simulink model "thermal_subsystem_closed_loop_harness"  (R2023a)
settings: Solver=VariableStepAuto  StartTime=0.0  StopTime=600  RelTol=1e-3
PostLoadFcn:
  | run('thermal_subsystem_parameters.m')
  | run('thermal_subsytem_harness_parameters.m')
values from neighbouring files (symbols this model uses):
  coolant_initial_temperature = 293.15    [thermal_model_parameters.m]    (also in thermal_plant_h2f175_parameters.m)
undefined symbols (not defined in the file or in its folder): sigbuilder_block, stack
libraries: fl_lib x5, nesl_utility x3, simulink x1
settings Model: Creator=adrian.taveras  LastModifiedBy=stefan.notter
settings OptimizationCC: ReuseModelBlockBuffer=off

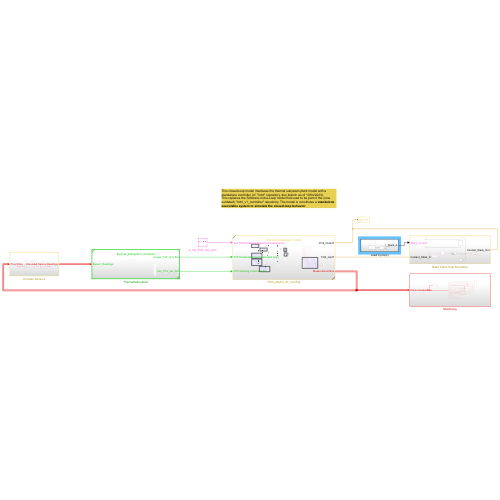
[thumbnail: Simulink's stored preview of the top-level diagram]
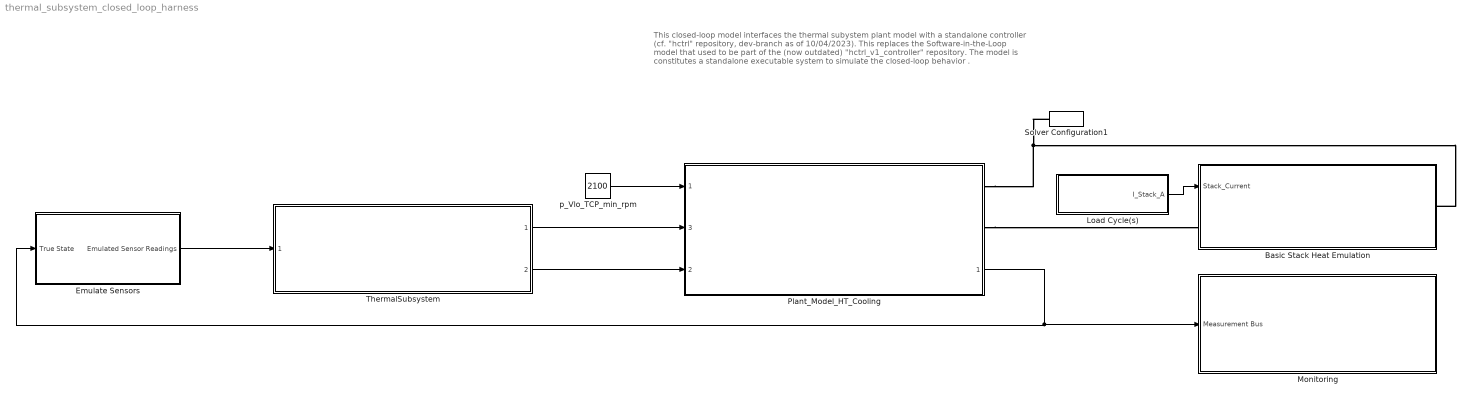
== system thermal_subsystem_closed_loop_harness ==
  note: This closed-loop model interfaces the thermal subystem plant model with a standalone controller (cf. "hctrl" repository, dev-branch as of 10/04/2023).
      | This replaces the Software-in-the-Loop model that used to be part of the (now outdated) "hctrl_v1_controller" repository. The model is constitutes a standalone executable system to simulate the closed-loop behavior .
  Basic Stack Heat Emulation : Subsystem
  Emulate Sensors : Subsystem
  Load Cycle(s) : Subsystem
  Monitoring : Subsystem
  Plant_Model_HT_Cooling : Subsystem  ReferencedSubsystem=thermal_subsystem_model
      settings: PortSchema="{\"entries\":[{\"content\":{\"sides\":[{\"content\":{\"connectorIds\":[\"Out1\",\"LConn1\",\"LConn2\"]},\"type\":\"ConnectorPlacement.EquallySpacedRectSide\",\"uuid\":\"706cf171-be05-45fb-992c-ba5e90f5cdb8\"},{\"content\":{\"connectorIds\":[\"In2\",\"In3\",\"In1\"],\"side\":\"RIGHT\"},\"type\":\"ConnectorPlacement.EquallySpacedRectSide\",\"uuid\":\"bf8ca14f-fef4-4eb5-a927-ccc799898aca\"},{\"content\":{\"side\":\"TOP\"},\"type\":\"ConnectorPlacement.EquallySpacedRectSide\",\"uuid\":\"9ad70fe7-ae85-4ea7-9728-0856e6ff40bf\"}]},\"type\":\"ConnectorPlacement.EquallySpacedConnector\",\"uuid\":\"91c985a6-7405-42c3-ac14-8c35e74d3001\"}],\"packageUris\":[\"http://schema.mathworks.com/mf0/Connector/R2020b\"],\"version\":\"1.0\"}"
  Solver Configuration1 : nesl_utility/Solver Configuration  PhysicalDomain=network_engine_domain  SubClassName=solver  LeftPortType=input  RightPortType=generic  Tones=[]  Harmonics=[]  SimulateNoise=off  Profile=off  UseLocalSampling=off  EnableSwitchedLinearOptims=on  FrequencyDomain=off  UseCCode=off  RelTol=0.001  AbsTol=1e-06  MinStep=1e-09  ToWorkspace=off  RevertToSquareIcSolve=off  NumHomotopyIterations=100  PhasorMode=off  PhasorModeNumHarmonics=1  ConsistencySolver=NEWTON_XTOL_AFTER_FTOL  IndexReductionMethod=DerivativeReplacement  DoDC=off  ResidualTolerance=1e-09  ConsistencyTolSource=GLOBAL  ConsistencyAbsTol=0.001  ConsistencyRelTol=0.001  ConsistencyTolFactor=0.001  UseLocalSolver=on  LocalSolverChoice=NE_BACKWARD_EULER_ADVANCER  ResolveIndetEquations=on  FunctionEvalNumThread=1  LocalSolverSampleTime=0.001  DoFixedCost=on  MaxNonlinIter=3  MaxModeIter=2  ComputeImpulses=off  ImpulseIterations=2  LinearAlgebra=auto  LinearAlgebraNumThread=0  EquationFormulation=NE_TIME_EF  DelaysMemoryBudget=1024  AutomaticFiltering=off  FilteringTimeConstant=0.001  PartitionStorageMethod=AS_NEEDED  PartitionMemoryBudget=1024  PartitionMethod=ROBUST
  ThermalSubsystem : Subsystem  TreatAsAtomicUnit=on  SystemSampleTime=0.02  ReferencedSubsystem=thermal_subsystem_controller
      settings: RTWFcnNameOpts=Use subsystem name  RTWFileNameOpts=Use subsystem name
  p_Vlo_TCP_min_rpm : Constant  Value=2100
  wires:
  Plant_Model_HT_Cooling/1 -> Emulate Sensors/1(True State), Monitoring/1(Measurement Bus)
  Emulate Sensors/1(Emulated Sensor Readings) -> ThermalSubsystem/1
  ThermalSubsystem/1 -> Plant_Model_HT_Cooling/3
  p_Vlo_TCP_min_rpm/1 -> Plant_Model_HT_Cooling/1
  ThermalSubsystem/2 -> Plant_Model_HT_Cooling/2
  Load Cycle(s)/1(I_Stack_A) -> Basic Stack Heat Emulation/1(Stack_Current)
  connections:
  Plant_Model_HT_Cooling/LConn1 -- Basic Stack Heat Emulation/LConn1
  Plant_Model_HT_Cooling/LConn2 -- Solver Configuration1/RConn1 -- Basic Stack Heat Emulation/RConn1

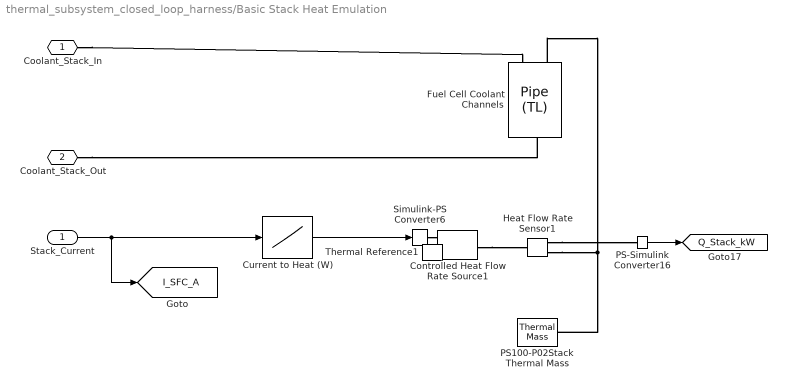
== system thermal_subsystem_closed_loop_harness/Basic Stack Heat Emulation ==
  Stack_Current : Inport
  Controlled Heat Flow Rate Source1 : fl_lib/Thermal/Thermal Sources/Controlled Heat Flow Rate Source
  Current to Heat (W) : Lookup_n-D  NumberOfTableDimensions=1  BreakpointsForDimension1=[0:50:400]  Table=[0, 9932, 21438, 33442,47123, 59491, 77033, 93585, 112042]  InternalRulePriority=Speed  RndMeth=Simplest
  Fuel Cell Coolant Channels : fl_lib/Thermal Liquid/Elements/Pipe (TL)  length=sqrt(stack.area) * stack.coolant_num_passes cm  area=stack.coolant_w_channels^2 * stack.coolant_num_layers cm^2  Dh=stack.coolant_w_channels cm  length_add=10 cm  roughness=15e-5 m  Re_lam=2000  Re_tur=4000  shape_factor=64  Nu_lam=3.66  dynamic_compressibility=simscape.enum.onoff.on  inertia=simscape.enum.onoff.off  p0=coolant_initial_pressure MPa  T0=coolant_initial_temperature K  mdot0=0 kg/s
  Heat Flow Rate Sensor1 : fl_lib/Thermal/Thermal Sensors/Heat Flow Rate Sensor
  PS-Simulink Converter16 : nesl_utility/PS-Simulink Converter  PhysicalDomain=network_engine_domain  SubClassName=ps_output  LeftPortType=input  RightPortType=output  PseudoPeriodic=off  Frequencies=[]  VectorFormat=1-D array  Unit=kW  AffineConversion=off
  PS100-P02Stack Thermal Mass : fl_lib/Thermal/Thermal Elements/Thermal Mass  mass_type=foundation.enum.constant_variable.constant  mass=stack.thermal_mass kg  sp_heat=stack.specific_heat J/kg/K  mass_min=1e-6 kg  num_ports=foundation.enum.numPorts2.one  m_specify=off  m_priority=High  m=1 kg  m_nominal_specify=off  m_nominal_unit=kg  m_nominal_value=1  T_specify=on  T_priority=High  T=coolant_initial_temperature K  T_nominal_specify=off  T_nominal_unit=K  T_nominal_value=1  Q_specify=off  Q_priority=None  Q=20e3 W  Q_nominal_specify=off  Q_nominal_unit=W  Q_nominal_value=1
  Simulink-PS Converter6 : nesl_utility/Simulink-PS Converter  PhysicalDomain=network_engine_domain  SubClassName=ps_input  LeftPortType=input  RightPortType=output  PseudoPeriodic=off  Frequencies=[]  NoiseDistribution=none  NoiseParameters=[]  Unit=J/s  AffineConversion=off  FilteringAndDerivatives=provide  SimscapeFilterOrder=1  InputFilterTimeConstant=0.001  UdotUserProvided=0
  Thermal Reference1 : fl_lib/Thermal/Thermal Elements/Thermal Reference
  Coolant_Stack_Out : PMIOPort  Port=2  Side=Right
  Coolant_Stack_In : PMIOPort  Side=Left
  tag scope: I_SFC_A=global, Q_Stack_kW=global
  wires:
  Current to Heat (W)/1 -> Simulink-PS Converter6/1
  PS-Simulink Converter16/1 -> [Q_Stack_kW]
  Stack_Current/1 -> Current to Heat (W)/1, [I_SFC_A]
  connections:
  Thermal Reference1/LConn1 -- Controlled Heat Flow Rate Source1/RConn2
  Controlled Heat Flow Rate Source1/LConn1 -- Heat Flow Rate Sensor1/LConn1
  Fuel Cell Coolant Channels/LConn2 -- Heat Flow Rate Sensor1/RConn2 -- PS100-P02Stack Thermal Mass/LConn1
  Heat Flow Rate Sensor1/RConn1 -- PS-Simulink Converter16/LConn1
  Simulink-PS Converter6/RConn1 -- Controlled Heat Flow Rate Source1/RConn1
  Coolant_Stack_In/RConn1 -- Fuel Cell Coolant Channels/LConn1
  Coolant_Stack_Out/RConn1 -- Fuel Cell Coolant Channels/RConn1

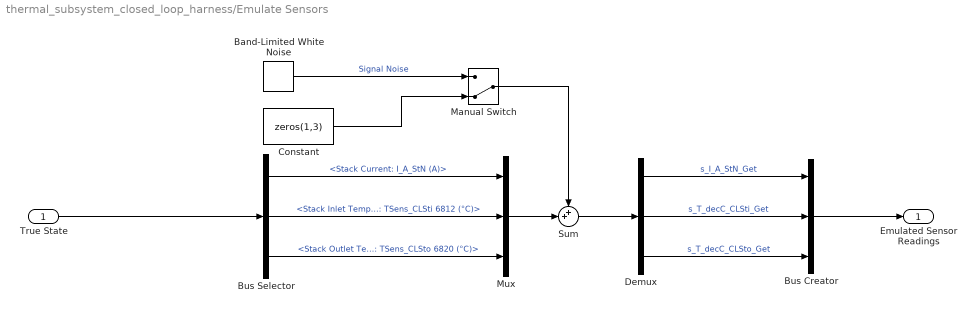
== system thermal_subsystem_closed_loop_harness/Emulate Sensors ==
  True State : Inport
  Band-Limited White Noise : simulink/Sources/Band-Limited White Noise  Cov=[5e-3, 5e-4, 5e-4]  Ts=0.1  seed=[23341]
  Bus Creator : BusCreator  Inputs=3
  Bus Selector : BusSelector  OutputSignals=Stack Current: I_A_StN (A),Stack Inlet Temperature: TSens_CLSti 6812 (°C),Stack Outlet Temperature: TSens_CLSto 6820 (°C)
  Constant : Constant  Value=zeros(1,3)
  Demux : Demux  Outputs=3
  Manual Switch : ManualSwitch  CurrentSetting=0
  Mux : Mux  Inputs=3
  Sum : Sum  Inputs=++|
  Emulated Sensor Readings : Outport
  wires:
  Bus Creator/1 -> Emulated Sensor Readings/1
  True State/1 -> Bus Selector/1
  Bus Selector/1 -> Mux/1  "<Stack Current: I_A_StN (A)>"
  Bus Selector/2 -> Mux/2  "<Stack Inlet Temperature: TSens_CLSti 6812 (°C)>"
  Bus Selector/3 -> Mux/3  "<Stack Outlet Temperature: TSens_CLSto 6820 (°C)>"
  Mux/1 -> Sum/2
  Sum/1 -> Demux/1
  Manual Switch/1 -> Sum/1
  Band-Limited White Noise/1 -> Manual Switch/1  "Signal Noise"
  Constant/1 -> Manual Switch/2
  Demux/1 -> Bus Creator/1  "s_I_A_StN_Get"
  Demux/3 -> Bus Creator/3  "s_T_decC_CLSto_Get"
  Demux/2 -> Bus Creator/2  "s_T_decC_CLSti_Get"

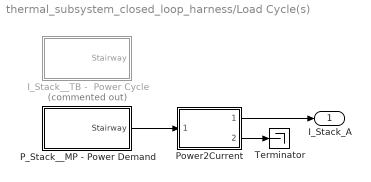
== system thermal_subsystem_closed_loop_harness/Load Cycle(s) ==
  I_Stack__TB -  Power Cycle : Subsystem  Tag=STV Subsys  Commented=on  LoadFcn=sigbuilder_block('load');  StartFcn=sigbuilder_block('start');  StopFcn=sigbuilder_block('stop');  ClipboardFcn=sigbuilder_block('clipboard');  mask(Sigbuilder block){tuvar=[0:10]}
      mask help: Simulink:masks:SigbuilderBlock_MD
      mask init:
      | if ~strcmp(get_param(bdroot(gcbh),'SimulationStatus'),'stopped') tuvar = sigbuilder_block('maskInit'); end
      settings: CopyFcn=sigbuilder_block('copy');  DeleteFcn=sigbuilder_block('delete');  ModelCloseFcn=sigbuilder_block('modelClose');  PreSaveFcn=sigbuilder_block('preSave');  PauseFcn=sigbuilder_block('pause');  ContinueFcn=sigbuilder_block('continue');  NameChangeFcn=sigbuilder_block('namechange');  OpenFcn=sigbuilder_block('open',[150.6 139.8 551.4 322.2 ]);  CloseFcn=sigbuilder_block('close');
      mask Display: plot(0, 0, 100, 100,[2, 2, 32, 32, 2], [68, 8, 8, 68, 68],[32, 2], [38, 38], [32, 19, 2],[53, 60, 44], [32, 17, 17, 2],[16, 16, 31, 31]);txt = getActiveGroup(gcbh);text(2, 100, txt,'verticalAlignment', 'top');
  P_Stack__MP - Power Demand : Subsystem  Tag=STV Subsys  LoadFcn=sigbuilder_block('load');  StartFcn=sigbuilder_block('start');  StopFcn=sigbuilder_block('stop');  ClipboardFcn=sigbuilder_block('clipboard');  mask(Sigbuilder block){tuvar=[0:10]}
      mask help: Simulink:masks:SigbuilderBlock_MD
      mask init:
      | if ~strcmp(get_param(bdroot(gcbh),'SimulationStatus'),'stopped') tuvar = sigbuilder_block('maskInit'); end
      settings: CopyFcn=sigbuilder_block('copy');  DeleteFcn=sigbuilder_block('delete');  ModelCloseFcn=sigbuilder_block('modelClose');  PreSaveFcn=sigbuilder_block('preSave');  PauseFcn=sigbuilder_block('pause');  ContinueFcn=sigbuilder_block('continue');  NameChangeFcn=sigbuilder_block('namechange');  OpenFcn=sigbuilder_block('open',[5.4 5.4 1141.2 580.8 ]);  CloseFcn=sigbuilder_block('close');
      mask Display: plot(0, 0, 100, 100,[2, 2, 32, 32, 2], [68, 8, 8, 68, 68],[32, 2], [38, 38], [32, 19, 2],[53, 60, 44], [32, 17, 17, 2],[16, 16, 31, 31]);txt = getActiveGroup(gcbh);text(2, 100, txt,'verticalAlignment', 'top');
  Power2Current : Subsystem
  Terminator : Terminator
  I_Stack_A : Outport
  wires:
  P_Stack__MP - Power Demand/1(Stairway) -> Power2Current/1(P_Stack)
  Power2Current/2(V_Stack) -> Terminator/1
  Power2Current/1(I_Stack) -> I_Stack_A/1

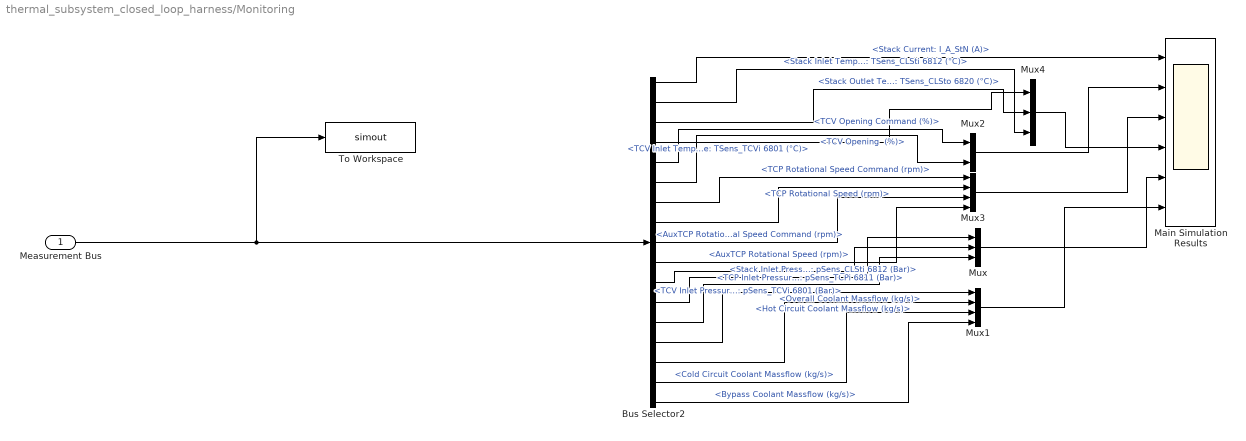
== system thermal_subsystem_closed_loop_harness/Monitoring ==
  Measurement Bus : Inport
  Bus Selector2 : BusSelector  OutputSignals="Stack Current: I_A_StN (A),Stack Inlet Temperature: TSens_CLSti 6812 (°C),Stack Outlet Temperature: TSens_CLSto 6820 (°C),TCV Inlet Temperature: TSens_TCVi 6801 (°C),TCV Opening Command (%),TCV Opening  (%),TCP Rotational Speed Command (rpm),TCP Rotational Speed (rpm),AuxTCP Rotational Speed Command (rpm),AuxTCP Rotational Speed (rpm),TCP Inlet Pressure: pSens_TCPi 6811 (Bar),Stack Inlet Pressure: pSens_CLSti 6812 (Bar),TCV Inlet Pressure: pSens_TCVi 6801 (Bar),Overall Coolant Massflow (kg/s),Hot Circuit Coolant Massflow (kg/s),Cold Circuit Coolant Massflow (kg/s),Bypass Coolant Massflow (kg/s)"
  Main Simulation Results : Scope  NumInputPorts=6
  Mux : Mux  Inputs=3
  Mux1 : Mux
  Mux2 : Mux  Inputs=2
  Mux3 : Mux
  Mux4 : Mux  Inputs=3
  To Workspace : ToWorkspace  VariableName=simout  SaveFormat=Timeseries  SampleTime=-1
  wires:
  Bus Selector2/10 -> Mux3/4  "<AuxTCP Rotational Speed (rpm)>"
  Mux4/1 -> Main Simulation Results/4
  Bus Selector2/11 -> Mux/2  "<TCP Inlet Pressure: pSens_TCPi 6811 (Bar)>"
  Mux3/1 -> Main Simulation Results/3
  Bus Selector2/7 -> Mux3/1  "<TCP Rotational Speed Command (rpm)>"
  Bus Selector2/3 -> Mux4/2  "<Stack Outlet Temperature: TSens_CLSto 6820 (°C)>"
  Mux2/1 -> Main Simulation Results/2
  Measurement Bus/1 -> To Workspace/1, Bus Selector2/1
  Bus Selector2/9 -> Mux3/3  "<AuxTCP Rotational Speed Command (rpm)>"
  Bus Selector2/2 -> Mux4/3  "<Stack Inlet Temperature: TSens_CLSti 6812 (°C)>"
  Bus Selector2/6 -> Mux2/2  "<TCV Opening  (%)>"
  Mux/1 -> Main Simulation Results/5
  Bus Selector2/15 -> Mux1/2  "<Hot Circuit Coolant Massflow (kg/s)>"
  Bus Selector2/13 -> Mux/3  "<TCV Inlet Pressure: pSens_TCVi 6801 (Bar)>"
  Bus Selector2/14 -> Mux1/1  "<Overall Coolant Massflow (kg/s)>"
  Mux1/1 -> Main Simulation Results/6
  Bus Selector2/17 -> Mux1/4  "<Bypass Coolant Massflow (kg/s)>"
  Bus Selector2/8 -> Mux3/2  "<TCP Rotational Speed (rpm)>"
  Bus Selector2/5 -> Mux2/1  "<TCV Opening Command (%)>"
  Bus Selector2/16 -> Mux1/3  "<Cold Circuit Coolant Massflow (kg/s)>"
  Bus Selector2/12 -> Mux/1  "<Stack Inlet Pressure: pSens_CLSti 6812 (Bar)>"
  Bus Selector2/4 -> Mux4/1  "<TCV Inlet Temperature: TSens_TCVi 6801 (°C)>"
  Bus Selector2/1 -> Main Simulation Results/1  "<Stack Current: I_A_StN (A)>"

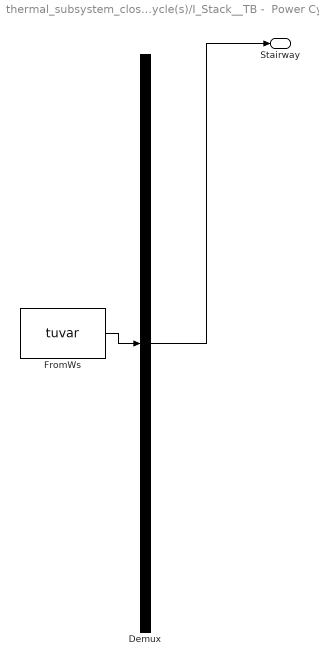
== system thermal_subsystem_closed_loop_harness/Load Cycle(s)/I_Stack__TB -  Power Cycle ==
  Demux : Demux  Tag=STV Demux  Outputs=1
      settings: DisplayOption=none
  FromWs : FromWorkspace  Tag=STV FromWs  VariableName=tuvar
      SigBuilderData=|
      | common.afterFinalStr = 'Extrapolate'
      | common.sampleTime = 0
      | dataSet.timeRange = [0 600]
      | dataSet.name = 'Group 1'
      | sbobj.Groups.Name = 'Group 1'
      | sbobj.Groups.Signals.Name = 'Stairway'
      | sbobj.Groups.Signals.XData = [0 180 190 250 260 320 330 390 400 460 470 530 540 600]
      | sbobj.Groups.Signals.YData = [100 100 200 200 300 300 400 400 300 300 200 200 100 100]
      | sbobj.Groups.TimeRange = [0 600]
  Stairway : Outport  Tag=STV Outport
  wires:
  Demux/1 -> Stairway/1
  FromWs/1 -> Demux/1

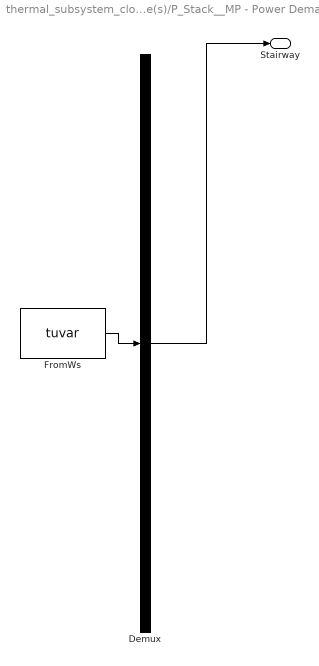
== system thermal_subsystem_closed_loop_harness/Load Cycle(s)/P_Stack__MP - Power Demand ==
  Demux : Demux  Tag=STV Demux  Outputs=1
      settings: DisplayOption=none
  FromWs : FromWorkspace  Tag=STV FromWs  VariableName=tuvar
      SigBuilderData=|
      | common.afterFinalStr = 'Extrapolate'
      | common.sampleTime = 0
      | dataSet.timeRange = [0 22226]
      | dataSet.name = 'Group 1'
      | sbobj.Groups.Name = 'Group 1'
      | sbobj.Groups.Signals.Name = 'Stairway'
      | sbobj.Groups.Signals.XData = [0 1 1.1 1.2 1.3 60 120 5000 5000 21146 21826 22226]
      | sbobj.Groups.Signals.YData = [0 0 0 0 1 1 100 100 85 85 25 1]
      | sbobj.Groups.TimeRange = [0 22226]
  Stairway : Outport  Tag=STV Outport
  wires:
  FromWs/1 -> Demux/1
  Demux/1 -> Stairway/1

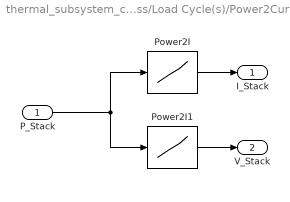
== system thermal_subsystem_closed_loop_harness/Load Cycle(s)/Power2Current ==
  P_Stack : Inport
  Power2I : Lookup_n-D  NumberOfTableDimensions=1  BreakpointsForDimension1=[0;8.5;17;26;34;42;50;58.3;66.66;85;100]  Table=[0;50;100;150;200;250;300;350;400;510;600]  InternalRulePriority=Speed  RndMeth=Simplest
  Power2I1 : Lookup_n-D  NumberOfTableDimensions=1  BreakpointsForDimension1=[0;8.5;17;26;34;42;50;58.3;66.66;85;100]  Table=[370;350;330;310;290;270;250;226;210;186;166.66]  InternalRulePriority=Speed  RndMeth=Simplest
  I_Stack : Outport
  V_Stack : Outport  Port=2
  wires:
  P_Stack/1 -> Power2I1/1, Power2I/1
  Power2I/1 -> I_Stack/1
  Power2I1/1 -> V_Stack/1
